simulink model "sampleModel1997"  (R2023a)
settings: Solver=VariableStepAuto  StartTime=0.0  StopTime=10.0  RelTol=1e-3
libraries: hdlsllib x3, simulink x3
settings Model: Creator=user1  LastModifiedBy=user1

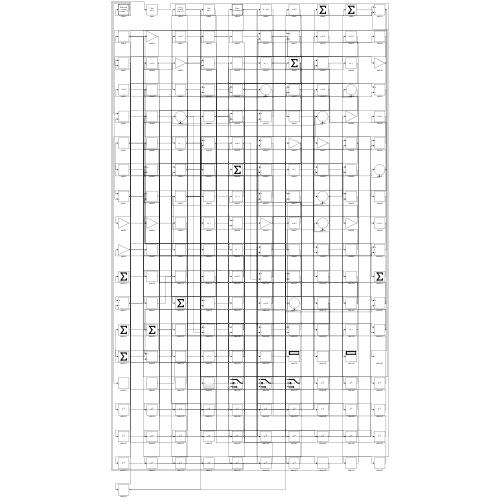
[thumbnail: Simulink's stored preview of the top-level diagram]
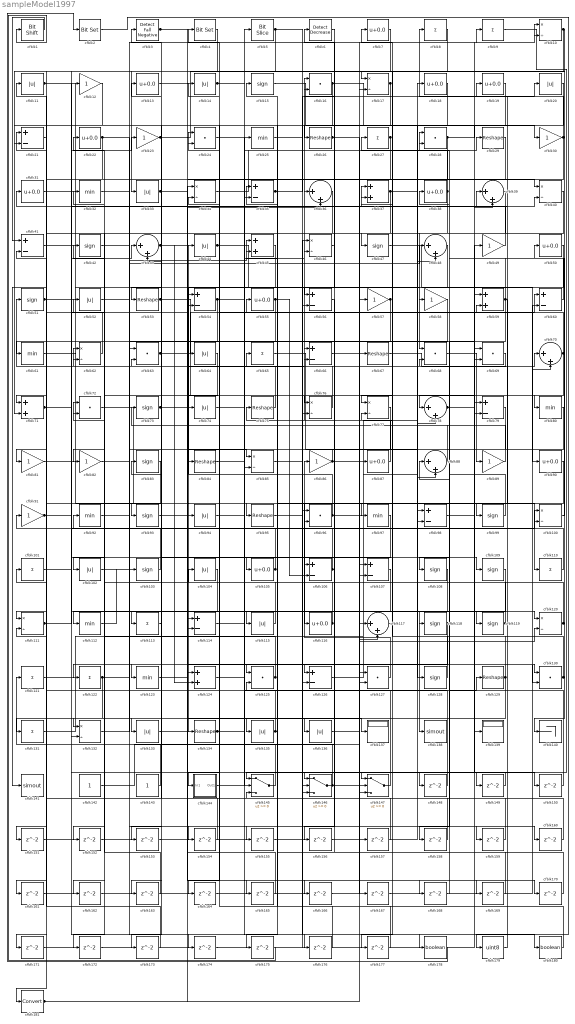
== system sampleModel1997 ==
  cfblk1 : hdlsllib/Logic and Bit Operations/Bit Shift  mode=Shift Left Logical  N=0
  cfblk{10,17,34,40,46,62,76..77,85,100,111,120,132} (13 alike) : Product  Inputs=*/  RndMeth=Zero  SaturateOnIntegerOverflow=on
  cfblk{8..9,27,65,101,110,113,121..122,131} (10 alike) : Sum  Inputs=+
  cfblk{11,14,20,33,44,52,64,74,94,102,104,115,133,135..136} (15 alike) : Abs  SaturateOnIntegerOverflow=off
  cfblk{15,42,47,51,73,83,93,99,103,108..109,118..119,128} (14 alike) : Signum
  cfblk{7,13,18..19,22,31,38,50,55,87,90,105,116} (13 alike) : Bias  Bias=0.0  SaturateOnIntegerOverflow=off
  cfblk{21,35,41,54,56,60,66,79,98,106..107,114,126} (13 alike) : Sum  Inputs=+-
  cfblk{25,32,61,80,92,97,112,123} (8 alike) : MinMax
  cfblk{36,39,43,48,70,78,88,117} (8 alike) : Sum  Inputs=|++
  cfblk{12,23,30,49,57..58,81..82,86,89,91} (11 alike) : Gain
  cfblk{37,45,59,71,124} (5 alike) : Sum
  cfblk{16,24,28,63,68..69,72,96,125,127,130} (11 alike) : DotProduct  OutDataTypeStr=Inherit: Inherit via internal rule
  cfblk{26,29,53,67,75,84,95,129,134} (9 alike) : Reshape
  cfblk137 : Display
  cfblk138 : ToWorkspace  VariableName=simout  SaveFormat=Timeseries  SampleTime=-1
  cfblk139 : Display
  cfblk140 : Terminator
  cfblk141 : ToWorkspace  VariableName=simout  SaveFormat=Timeseries  SampleTime=-1
  cfblk142 : Constant  SampleTime=-1
  cfblk143 : Constant  SampleTime=-1
  cfblk144 : Subsystem
      settings: LibrarySourceBlock=|
      | hdlsllib/Ports &
      | Subsystems/Subsystem
  cfblk145 : Switch  SaturateOnIntegerOverflow=off  InputSameDT=off
  cfblk146 : Switch  SaturateOnIntegerOverflow=off  InputSameDT=off
  cfblk147 : Switch  SaturateOnIntegerOverflow=off  InputSameDT=off
  cfblk{148..177} (30 alike) : Delay  SampleTime=1
  cfblk178 : DataTypeConversion  OutDataTypeStr=boolean  SaturateOnIntegerOverflow=off  RndMeth=Floor
  cfblk179 : DataTypeConversion  OutDataTypeStr=uint8  SaturateOnIntegerOverflow=off  RndMeth=Floor
  cfblk180 : DataTypeConversion  OutDataTypeStr=boolean  SaturateOnIntegerOverflow=off  RndMeth=Floor
  cfblk181 : DataTypeConversion  SaturateOnIntegerOverflow=off  RndMeth=Floor
  cfblk2 : simulink/Logic and Bit Operations/Bit Set  iBit=0
      settings: LibrarySourceBlock=|
      | hdlsllib/Logic and Bit
      | Operations/Bit Set
  cfblk3 : hdlsllib/Logic and Bit Operations/Detect Fall Negative  vinit=0  OutDataTypeStr=boolean
  cfblk4 : simulink/Logic and Bit Operations/Bit Set  iBit=0
      settings: LibrarySourceBlock=|
      | hdlsllib/Logic and Bit
      | Operations/Bit Set
  cfblk5 : hdlsllib/Logic and Bit Operations/Bit Slice  lidx=7  ridx=0
  cfblk6 : simulink/Logic and Bit Operations/Detect Decrease  vinit=0.0  OutDataTypeStr=boolean
      settings: LibrarySourceBlock=|
      | hdlsllib/Logic and Bit
      | Operations/Detect
      | Decrease
  wires:
  cfblk70/1 -> cfblk78/1, cfblk24/2
  cfblk34/1 -> cfblk29/1
  cfblk50/1 -> cfblk134/1
  cfblk76/1 -> cfblk51/1
  cfblk43/1 -> cfblk124/2, cfblk148/1
  cfblk133/1 -> cfblk37/1
  cfblk77/1 -> cfblk121/1
  cfblk112/1 -> cfblk103/1
  cfblk62/1 -> cfblk141/1
  cfblk31/1 -> cfblk95/1
  cfblk15/1 -> cfblk30/1
  cfblk103/1 -> cfblk92/1
  cfblk94/1 -> cfblk25/1
  cfblk108/1 -> cfblk138/1
  cfblk23/1 -> cfblk140/1, cfblk79/2
  cfblk9/1 -> cfblk147/1
  cfblk29/1 -> cfblk144/1(In1)
  cfblk127/1 -> cfblk86/1
  cfblk51/1 -> cfblk116/1, cfblk174/1
  cfblk61/1 -> cfblk94/1
  cfblk8/1 -> cfblk77/1
  cfblk18/1 -> cfblk47/1
  cfblk17/1 -> cfblk125/1, cfblk114/1
  cfblk147/1 -> cfblk101/1
  cfblk96/1 -> cfblk44/1, cfblk18/1
  cfblk3/1 -> cfblk40/1, cfblk97/1
  cfblk91/1 -> cfblk40/2, cfblk114/2
  cfblk33/1 -> cfblk133/1, cfblk126/1
  cfblk11/1 -> cfblk110/1, cfblk146/3, cfblk109/1
  cfblk55/1 -> cfblk102/1, cfblk106/2
  cfblk129/1 -> cfblk131/1, cfblk91/1
  cfblk60/1 -> cfblk27/1
  cfblk104/1 -> cfblk112/1
  cfblk126/1 -> cfblk60/1
  cfblk68/1 -> cfblk89/1
  cfblk99/1 -> cfblk31/1
  cfblk125/1 -> cfblk72/1, cfblk123/1
  cfblk111/1 -> cfblk43/1, cfblk100/2
  cfblk110/1 -> cfblk65/1
  cfblk16/1 -> cfblk139/1, cfblk88/2, cfblk171/1
  cfblk49/1 -> cfblk16/1
  cfblk7/1 -> cfblk33/1
  cfblk1/1 -> cfblk41/1
  cfblk46/1 -> cfblk6/1
  cfblk19/1 -> cfblk53/1
  cfblk86/1 -> cfblk84/1, cfblk120/1
  cfblk87/1 -> cfblk36/1
  cfblk100/1 -> cfblk50/1
  cfblk63/1 -> cfblk55/1, cfblk130/2
  cfblk131/1 -> cfblk100/1
  cfblk40/1 -> cfblk68/1
  cfblk37/1 -> cfblk98/1, cfblk82/1
  cfblk101/1 -> cfblk12/1
  cfblk52/1 -> cfblk69/2
  cfblk44/1 -> cfblk127/2, cfblk28/1, cfblk46/2
  cfblk39/1 -> cfblk98/2
  cfblk56/1 -> cfblk146/1
  cfblk75/1 -> cfblk11/1
  cfblk109/1 -> cfblk113/1
  cfblk78/1 -> cfblk49/1, cfblk108/1
  cfblk142/1 -> cfblk87/1
  cfblk30/1 -> cfblk8/1, cfblk177/1
  cfblk69/1 -> cfblk63/2
  cfblk120/1 -> cfblk32/1, cfblk34/2
  cfblk81/1 -> cfblk93/1
  cfblk10/1 -> cfblk80/1, cfblk132/2
  cfblk130/1 -> cfblk75/1, cfblk39/1
  cfblk6/1 -> cfblk26/1
  cfblk32/1 -> cfblk85/1
  cfblk128/1 -> cfblk37/2
  cfblk38/1 -> cfblk61/1, cfblk28/2, cfblk163/1
  cfblk22/1 -> cfblk111/1, cfblk176/1
  cfblk42/1 -> cfblk115/1
  cfblk88/1 -> cfblk7/1
  cfblk143/1 -> cfblk21/1
  cfblk65/1 -> cfblk128/1
  cfblk35/1 -> cfblk20/1, cfblk170/1
  cfblk121/1 -> cfblk67/1
  cfblk27/1 -> cfblk135/1, cfblk35/2, cfblk71/1
  cfblk115/1 -> cfblk14/1
  cfblk4/1 -> cfblk181/1
  cfblk106/1 -> cfblk3/1, cfblk66/1
  cfblk58/1 -> cfblk105/1
  cfblk72/1 -> cfblk117/1
  cfblk67/1 -> cfblk70/1
  cfblk135/1 -> cfblk83/1, cfblk35/1
  cfblk5/1 -> cfblk17/1, cfblk71/2, cfblk149/1
  cfblk124/1 -> cfblk96/2
  cfblk21/1 -> cfblk81/1
  cfblk132/1 -> cfblk45/1
  cfblk41/1 -> cfblk58/1
  cfblk26/1 -> cfblk118/1, cfblk10/2
  cfblk144/1(Out1) -> cfblk129/1
  cfblk12/1 -> cfblk21/2
  cfblk145/1 -> cfblk22/1
  cfblk119/1 -> cfblk24/1, cfblk62/2
  cfblk93/1 -> cfblk137/1
  cfblk48/1 -> cfblk107/2
  cfblk92/1 -> cfblk119/1
  cfblk146/1 -> cfblk45/2, cfblk120/2
  cfblk47/1 -> cfblk90/1
  cfblk116/1 -> cfblk42/1, cfblk106/1
  cfblk14/1 -> cfblk5/1, cfblk39/2
  cfblk53/1 -> cfblk76/1, cfblk79/1
  cfblk59/1 -> cfblk99/1, cfblk38/1, cfblk158/1
  cfblk113/1 -> cfblk13/1
  cfblk79/1 -> cfblk85/2
  cfblk54/1 -> cfblk147/2, cfblk162/1
  cfblk57/1 -> cfblk74/1, cfblk161/1
  cfblk102/1 -> cfblk48/1
  cfblk20/1 -> cfblk56/1
  cfblk82/1 -> cfblk9/1
  cfblk117/1 -> cfblk77/2
  cfblk89/1 -> cfblk73/1
  cfblk24/1 -> cfblk136/1
  cfblk45/1 -> cfblk64/1
  cfblk122/1 -> cfblk132/1, cfblk154/1, cfblk155/1
  cfblk134/1 -> cfblk104/1, cfblk59/2
  cfblk85/1 -> cfblk46/1
  cfblk118/1 -> cfblk122/1, cfblk153/1
  cfblk73/1 -> cfblk147/3, cfblk66/2, cfblk165/1, cfblk166/1, cfblk168/1
  cfblk107/1 -> cfblk145/2
  cfblk105/1 -> cfblk62/1, cfblk52/1
  cfblk13/1 -> cfblk36/2
  cfblk28/1 -> cfblk10/1, cfblk164/1
  cfblk71/1 -> cfblk23/1, cfblk54/2
  cfblk123/1 -> cfblk130/1
  cfblk148/1 -> cfblk63/1
  cfblk149/1 -> cfblk145/1
  cfblk98/1 -> cfblk150/1
  cfblk150/1 -> cfblk88/1
  cfblk83/1 -> cfblk151/1
  cfblk151/1 -> cfblk78/2
  cfblk64/1 -> cfblk152/1
  cfblk152/1 -> cfblk127/1
  cfblk153/1 -> cfblk146/2
  cfblk154/1 -> cfblk41/2
  cfblk155/1 -> cfblk48/2
  cfblk80/1 -> cfblk156/1
  cfblk156/1 -> cfblk107/1
  cfblk136/1 -> cfblk157/1
  cfblk157/1 -> cfblk124/1
  cfblk158/1 -> cfblk43/2
  cfblk95/1 -> cfblk159/1
  cfblk159/1 -> cfblk59/1
  cfblk74/1 -> cfblk160/1
  cfblk160/1 -> cfblk96/1
  cfblk161/1 -> cfblk56/2
  cfblk162/1 -> cfblk60/2
  cfblk163/1 -> cfblk72/2
  cfblk164/1 -> cfblk126/2
  cfblk165/1 -> cfblk34/1
  cfblk166/1 -> cfblk17/2
  cfblk66/1 -> cfblk167/1
  cfblk167/1 -> cfblk70/2
  cfblk168/1 -> cfblk68/2
  cfblk114/1 -> cfblk169/1
  cfblk169/1 -> cfblk125/2
  cfblk170/1 -> cfblk16/2
  cfblk171/1 -> cfblk117/2
  cfblk36/1 -> cfblk172/1
  cfblk172/1 -> cfblk69/1
  cfblk97/1 -> cfblk173/1
  cfblk173/1 -> cfblk111/2
  cfblk174/1 -> cfblk76/2
  cfblk90/1 -> cfblk175/1
  cfblk175/1 -> cfblk1/1
  cfblk176/1 -> cfblk145/3
  cfblk177/1 -> cfblk15/1
  cfblk84/1 -> cfblk178/1
  cfblk178/1 -> cfblk2/1
  cfblk2/1 -> cfblk179/1
  cfblk179/1 -> cfblk19/1
  cfblk25/1 -> cfblk180/1
  cfblk180/1 -> cfblk4/1
  cfblk181/1 -> cfblk54/1, cfblk57/1

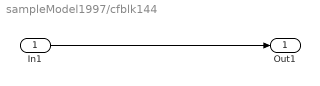
== system sampleModel1997/cfblk144 ==
  In1 : Inport
  Out1 : Outport
  wires:
  In1/1 -> Out1/1
